simulink model "decoder_modeli"  (R2021a)
settings: Solver=VariableStepAuto  StartTime=0.0  StopTime=0.0001  RelTol=1e-4
libraries: simulink_extras x18, simulink x2, commrandsrc3 x1, dsparch4 x1, dspswit3 x1
settings Model: Creator=Administrator  LastModifiedBy=Administrator
settings DebuggingCC: StringTruncationChecking=none  MultiTaskDSMMsg=none  ParameterDowncastMsg=none  ParameterOverflowMsg=none  ParameterPrecisionLossMsg=none  ParameterTunabilityLossMsg=none

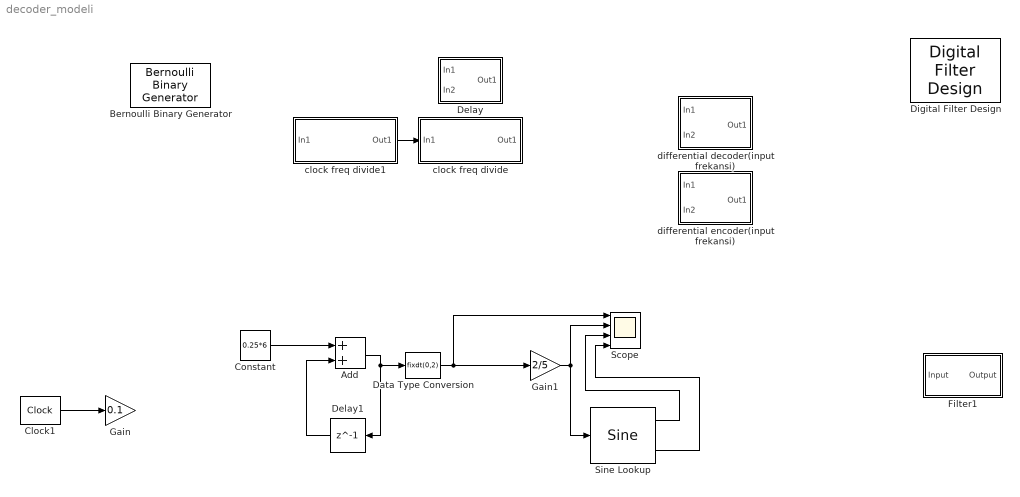
== system decoder_modeli ==
  Add : Sum  AccumDataTypeStr=double
  Bernoulli Binary Generator : commrandsrc3/Bernoulli Binary Generator  ProbabilityOfZero=0.5  SeedSource=Auto  Seed=12  SampleTime=1  SamplesPerFrame=1  OutputDataType=boolean  SimulateUsing=Interpreted execution
  Clock1 : simulink_extras/Flip Flops/Clock  period=1
  Constant : Constant  Value=0.25*6  OutDataTypeStr=double  SampleTime=25e-9
  Data Type Conversion : DataTypeConversion  OutMin=[0]  OutMax=[4]  OutDataTypeStr=fixdt(0,2)
  Delay : Subsystem
  Delay1 : Delay  DelayLength=1  InitialCondition=0  UseCircularBuffer=on  SampleTime=25e-9
  Digital Filter Design : dsparch4/Digital Filter Design  mwdsp_browser_bugfix_var=off
  Filter1 : Subsystem  Tag=FilterWizardSubSystem
      settings: ErrorFcn=dspFilterRealizedInBasicElemsAlgLoopErrFcnCallback
  Gain : Gain  Gain=0.1
  Gain1 : Gain  Gain=2/5
  Scope : Scope  NumInputPorts=4
  Sine Lookup : simulink/Lookup Tables/Sine  Formula=sin(2*pi*u) and cos(2*pi*u)  NumDataPoints=(2^1)+1  OutputWordLength=4  InternalRulePriority=Speed
  clock freq divide : Subsystem
  clock freq divide1 : Subsystem
  differential decoder(input frekansi) : Subsystem
  differential encoder(input frekansi) : Subsystem
  wires:
  clock freq divide1/1(Out1) -> clock freq divide/1(In1)
  Add/1 -> Delay1/1, Data Type Conversion/1
  Clock1/1 -> Gain/1
  Constant/1 -> Add/1
  Delay1/1 -> Add/2
  Sine Lookup/1 -> Scope/3
  Gain1/1 -> Scope/2, Sine Lookup/1
  Sine Lookup/2 -> Scope/4
  Data Type Conversion/1 -> Gain1/1, Scope/1

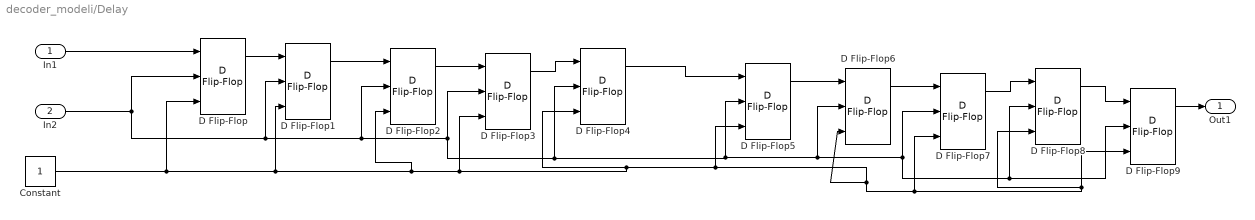
== system decoder_modeli/Delay ==
  In1 : Inport
  In2 : Inport  Port=2
  Constant : Constant
  D Flip-Flop{,1..9} (10 alike) : simulink_extras/Flip Flops/D Flip-Flop
  Out1 : Outport
  wires:
  D Flip-Flop/1 -> D Flip-Flop1/1
  In1/1 -> D Flip-Flop/1
  D Flip-Flop2/1 -> D Flip-Flop3/1
  D Flip-Flop1/1 -> D Flip-Flop2/1
  D Flip-Flop4/1 -> D Flip-Flop5/1
  D Flip-Flop3/1 -> D Flip-Flop4/1
  D Flip-Flop7/1 -> D Flip-Flop8/1
  D Flip-Flop6/1 -> D Flip-Flop7/1
  D Flip-Flop8/1 -> D Flip-Flop9/1
  Constant/1 -> D Flip-Flop9/3, D Flip-Flop8/3, D Flip-Flop7/3, D Flip-Flop6/3, D Flip-Flop5/3, D Flip-Flop4/3, D Flip-Flop3/3, D Flip-Flop2/3, D Flip-Flop1/3, D Flip-Flop/3
  In2/1 -> D Flip-Flop3/2, D Flip-Flop6/2, D Flip-Flop9/2, D Flip-Flop8/2, D Flip-Flop7/2, D Flip-Flop5/2, D Flip-Flop4/2, D Flip-Flop2/2, D Flip-Flop1/2, D Flip-Flop/2
  D Flip-Flop5/1 -> D Flip-Flop6/1
  D Flip-Flop9/1 -> Out1/1

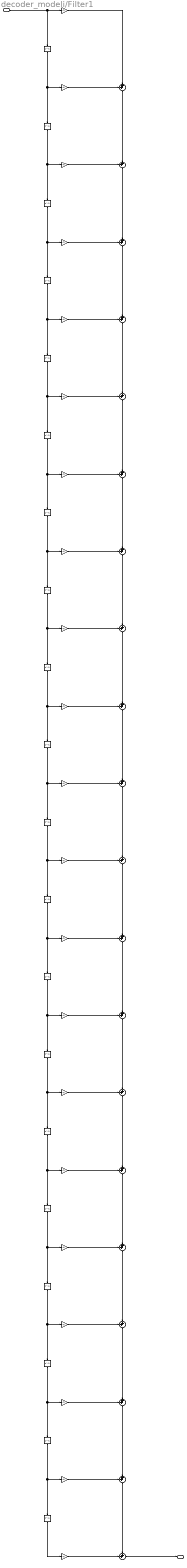
== system decoder_modeli/Filter1 ==
  Input : Inport
  BodyDelay{2..21} (20 alike) : Delay  DelayLength=1  InitialCondition=0  InputProcessing=Columns as channels (frame based)
  BodyLSum{2..21} (20 alike) : Sum  Inputs=++|  RndMeth=Nearest  SaturateOnIntegerOverflow=on  OutDataTypeStr=Inherit: Same as first input
  b(1) : Gain  Gain=3.69421067777138091e-19  ParamDataTypeStr=double  RndMeth=Nearest  SaturateOnIntegerOverflow=on  OutDataTypeStr=Inherit: Same as input
  b(10) : Gain  Gain=0.113897378800497842  ParamDataTypeStr=double  RndMeth=Nearest  SaturateOnIntegerOverflow=on  OutDataTypeStr=Inherit: Same as input
  b(11) : Gain  Gain=0.118459717673086246  ParamDataTypeStr=double  RndMeth=Nearest  SaturateOnIntegerOverflow=on  OutDataTypeStr=Inherit: Same as input
  b(12) : Gain  Gain=0.113897378800497842  ParamDataTypeStr=double  RndMeth=Nearest  SaturateOnIntegerOverflow=on  OutDataTypeStr=Inherit: Same as input
  b(13) : Gain  Gain=0.101082211156672042  ParamDataTypeStr=double  RndMeth=Nearest  SaturateOnIntegerOverflow=on  OutDataTypeStr=Inherit: Same as input
  b(14) : Gain  Gain=0.0824036741883590468  ParamDataTypeStr=double  RndMeth=Nearest  SaturateOnIntegerOverflow=on  OutDataTypeStr=Inherit: Same as input
  b(15) : Gain  Gain=0.0611569261162345293  ParamDataTypeStr=double  RndMeth=Nearest  SaturateOnIntegerOverflow=on  OutDataTypeStr=Inherit: Same as input
  b(16) : Gain  Gain=0.0407234511898747834  ParamDataTypeStr=double  RndMeth=Nearest  SaturateOnIntegerOverflow=on  OutDataTypeStr=Inherit: Same as input
  b(17) : Gain  Gain=0.0237792219561070405  ParamDataTypeStr=double  RndMeth=Nearest  SaturateOnIntegerOverflow=on  OutDataTypeStr=Inherit: Same as input
  b(18) : Gain  Gain=0.0117498026081423717  ParamDataTypeStr=double  RndMeth=Nearest  SaturateOnIntegerOverflow=on  OutDataTypeStr=Inherit: Same as input
  b(19) : Gain  Gain=0.00465025225065794634  ParamDataTypeStr=double  RndMeth=Nearest  SaturateOnIntegerOverflow=on  OutDataTypeStr=Inherit: Same as input
  b(2) : Gain  Gain=0.00132722289691133218  ParamDataTypeStr=double  RndMeth=Nearest  SaturateOnIntegerOverflow=on  OutDataTypeStr=Inherit: Same as input
  b(20) : Gain  Gain=0.00132722289691133218  ParamDataTypeStr=double  RndMeth=Nearest  SaturateOnIntegerOverflow=on  OutDataTypeStr=Inherit: Same as input
  b(21) : Gain  Gain=3.69421067777138091e-19  ParamDataTypeStr=double  RndMeth=Nearest  SaturateOnIntegerOverflow=on  OutDataTypeStr=Inherit: Same as input
  b(3) : Gain  Gain=0.00465025225065794634  ParamDataTypeStr=double  RndMeth=Nearest  SaturateOnIntegerOverflow=on  OutDataTypeStr=Inherit: Same as input
  b(4) : Gain  Gain=0.0117498026081423717  ParamDataTypeStr=double  RndMeth=Nearest  SaturateOnIntegerOverflow=on  OutDataTypeStr=Inherit: Same as input
  b(5) : Gain  Gain=0.0237792219561070405  ParamDataTypeStr=double  RndMeth=Nearest  SaturateOnIntegerOverflow=on  OutDataTypeStr=Inherit: Same as input
  b(6) : Gain  Gain=0.0407234511898747834  ParamDataTypeStr=double  RndMeth=Nearest  SaturateOnIntegerOverflow=on  OutDataTypeStr=Inherit: Same as input
  b(7) : Gain  Gain=0.0611569261162345293  ParamDataTypeStr=double  RndMeth=Nearest  SaturateOnIntegerOverflow=on  OutDataTypeStr=Inherit: Same as input
  b(8) : Gain  Gain=0.0824036741883590468  ParamDataTypeStr=double  RndMeth=Nearest  SaturateOnIntegerOverflow=on  OutDataTypeStr=Inherit: Same as input
  b(9) : Gain  Gain=0.101082211156672042  ParamDataTypeStr=double  RndMeth=Nearest  SaturateOnIntegerOverflow=on  OutDataTypeStr=Inherit: Same as input
  Output : Outport
  wires:
  Input/1 -> b(1)/1, BodyDelay2/1
  b(1)/1 -> BodyLSum2/2
  BodyDelay2/1 -> b(2)/1, BodyDelay3/1
  b(2)/1 -> BodyLSum2/1
  BodyLSum2/1 -> BodyLSum3/2
  BodyDelay3/1 -> b(3)/1, BodyDelay4/1
  b(3)/1 -> BodyLSum3/1
  BodyLSum3/1 -> BodyLSum4/2
  BodyDelay4/1 -> b(4)/1, BodyDelay5/1
  b(4)/1 -> BodyLSum4/1
  BodyLSum4/1 -> BodyLSum5/2
  BodyDelay5/1 -> b(5)/1, BodyDelay6/1
  b(5)/1 -> BodyLSum5/1
  BodyLSum5/1 -> BodyLSum6/2
  BodyDelay6/1 -> b(6)/1, BodyDelay7/1
  b(6)/1 -> BodyLSum6/1
  BodyLSum6/1 -> BodyLSum7/2
  BodyDelay7/1 -> b(7)/1, BodyDelay8/1
  b(7)/1 -> BodyLSum7/1
  BodyLSum7/1 -> BodyLSum8/2
  BodyDelay8/1 -> b(8)/1, BodyDelay9/1
  b(8)/1 -> BodyLSum8/1
  BodyLSum8/1 -> BodyLSum9/2
  BodyDelay9/1 -> b(9)/1, BodyDelay10/1
  b(9)/1 -> BodyLSum9/1
  BodyLSum9/1 -> BodyLSum10/2
  BodyDelay10/1 -> b(10)/1, BodyDelay11/1
  b(10)/1 -> BodyLSum10/1
  BodyLSum10/1 -> BodyLSum11/2
  BodyDelay11/1 -> b(11)/1, BodyDelay12/1
  b(11)/1 -> BodyLSum11/1
  BodyLSum11/1 -> BodyLSum12/2
  BodyDelay12/1 -> b(12)/1, BodyDelay13/1
  b(12)/1 -> BodyLSum12/1
  BodyLSum12/1 -> BodyLSum13/2
  BodyDelay13/1 -> b(13)/1, BodyDelay14/1
  b(13)/1 -> BodyLSum13/1
  BodyLSum13/1 -> BodyLSum14/2
  BodyDelay14/1 -> b(14)/1, BodyDelay15/1
  b(14)/1 -> BodyLSum14/1
  BodyLSum14/1 -> BodyLSum15/2
  BodyDelay15/1 -> b(15)/1, BodyDelay16/1
  b(15)/1 -> BodyLSum15/1
  BodyLSum15/1 -> BodyLSum16/2
  BodyDelay16/1 -> b(16)/1, BodyDelay17/1
  b(16)/1 -> BodyLSum16/1
  BodyLSum16/1 -> BodyLSum17/2
  BodyDelay17/1 -> b(17)/1, BodyDelay18/1
  b(17)/1 -> BodyLSum17/1
  BodyLSum17/1 -> BodyLSum18/2
  BodyDelay18/1 -> b(18)/1, BodyDelay19/1
  b(18)/1 -> BodyLSum18/1
  BodyLSum18/1 -> BodyLSum19/2
  BodyDelay19/1 -> b(19)/1, BodyDelay20/1
  b(19)/1 -> BodyLSum19/1
  BodyLSum19/1 -> BodyLSum20/2
  BodyDelay20/1 -> b(20)/1, BodyDelay21/1
  b(20)/1 -> BodyLSum20/1
  BodyLSum20/1 -> BodyLSum21/1
  BodyDelay21/1 -> b(21)/1
  b(21)/1 -> BodyLSum21/2
  BodyLSum21/1 -> Output/1

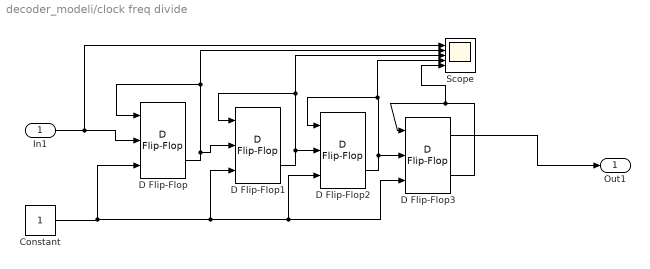
== system decoder_modeli/clock freq divide ==
  In1 : Inport
  Constant : Constant
  D Flip-Flop{,1..3} (4 alike) : simulink_extras/Flip Flops/D Flip-Flop
  Scope : Scope  NumInputPorts=5
  Out1 : Outport
  wires:
  D Flip-Flop/2 -> D Flip-Flop1/2, Scope/2, D Flip-Flop/1
  D Flip-Flop1/2 -> Scope/3, D Flip-Flop1/1, D Flip-Flop2/2
  D Flip-Flop3/2 -> Scope/5, D Flip-Flop3/1
  In1/1 -> Scope/1, D Flip-Flop/2
  Constant/1 -> D Flip-Flop3/3, D Flip-Flop2/3, D Flip-Flop1/3, D Flip-Flop/3
  D Flip-Flop3/1 -> Out1/1
  D Flip-Flop2/2 -> Scope/4, D Flip-Flop2/1, D Flip-Flop3/2

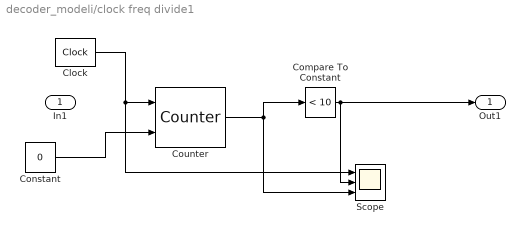
== system decoder_modeli/clock freq divide1 ==
  In1 : Inport
  Clock : simulink_extras/Flip Flops/Clock  period=2
  Compare To Constant : simulink/Logic and Bit Operations/Compare To Constant  relop=<  const=10  OutDataTypeStr=boolean
  Constant : Constant  Value=0
  Counter : dspswit3/Counter  Direction=Up  CountEvent=Rising edge  CounterSize=User defined  MaxCount=19  InitialCount=0  Output=Count  HitValue=19  ResetInput=on  SamplesPerFrame=1  Ts=1  CntDtype=int8  HitDtype=Logical
  Scope : Scope  NumInputPorts=3
  Out1 : Outport
  wires:
  Counter/1 -> Compare To Constant/1, Scope/3
  Clock/1 -> Scope/1, Counter/1
  Constant/1 -> Counter/2
  Compare To Constant/1 -> Scope/2, Out1/1

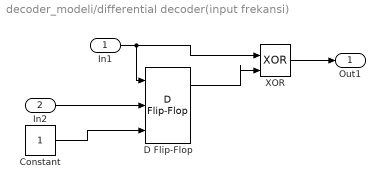
== system decoder_modeli/differential decoder(input frekansi) ==
  In1 : Inport
  In2 : Inport  Port=2
  Constant : Constant
  D Flip-Flop : simulink_extras/Flip Flops/D Flip-Flop
  XOR : Logic  Operator=XOR  IconShape=distinctive  AllPortsSameDT=off  OutDataTypeStr=boolean
  Out1 : Outport
  wires:
  D Flip-Flop/1 -> XOR/2
  XOR/1 -> Out1/1
  In2/1 -> D Flip-Flop/2
  In1/1 -> D Flip-Flop/1, XOR/1
  Constant/1 -> D Flip-Flop/3

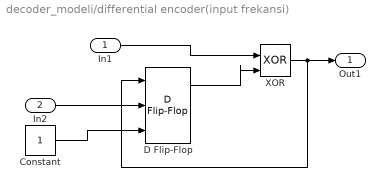
== system decoder_modeli/differential encoder(input frekansi) ==
  In1 : Inport
  In2 : Inport  Port=2
  Constant : Constant
  D Flip-Flop : simulink_extras/Flip Flops/D Flip-Flop
  XOR : Logic  Operator=XOR  IconShape=distinctive  AllPortsSameDT=off  OutDataTypeStr=boolean
  Out1 : Outport
  wires:
  D Flip-Flop/1 -> XOR/2
  In1/1 -> XOR/1
  In2/1 -> D Flip-Flop/2
  XOR/1 -> D Flip-Flop/1, Out1/1
  Constant/1 -> D Flip-Flop/3
